simulink model "HSP_TC499_Trajectory_Planning_Control"  (R2025a)
settings: Solver=FixedStepAuto  StartTime=0.0  StopTime=SIM_TIME  FixedStep=0.01  RelTol=1e-3  EnableMultiTasking=on
values from neighbouring files (symbols this model uses):
  D_COEFF = 2.631    [init_PID_controller.m]
  I_COEFF = 4.2108    [init_PID_controller.m]
  P_COEFF = 9.4365    [init_PID_controller.m]
settings Model: Creator=chmurski  LastModifiedBy=MarikL
settings SolverCC: PositivePriorityOrder=on  AutoInsertRateTranBlk=on
settings OptimizationCC: OptimizeBlockIOStorage=off  BufferReuse=off  ReuseModelBlockBuffer=off  GlobalBufferReuse=off  ExpressionFolding=off  EnableMemcpy=off  PassReuseOutputArgsAs=Individual arguments  LocalBlockOutputs=off  ZeroExternalMemoryAtStartup=off  ZeroInternalMemoryAtStartup=off  MaxStackSize=2048  OptimizeDataStoreBuffers=off  BusAssignmentInplaceUpdate=off  OptimizationLevel=level0  OptimizationCustomize=off  EfficientTunableParamExpr=on
settings DebuggingCC: ParameterTunabilityLossMsg=error
settings HardwareCC: ProdBitPerPointer=32.0  ProdBitPerSizeT=32.0  ProdBitPerPtrDiffT=32.0  ProdLargestAtomicInteger=Long  ProdWordSize=32.0  ProdLongLongMode=on  ProdHWDeviceType=Infineon->TriCore
settings SFSimCC: MATLABDynamicMemAlloc=off
settings RTWCC: SystemTargetFile=ert.tlc  HardwareBoard=Infineon AURIX TC4x - TriBoards  GenCodeOnly=on  PackageGeneratedCodeAndArtifacts=on  PackageName=packaged_code  TemplateMakefile=ert_default_tmf  Toolchain=TASKING SmartCode for TriCore  BuildConfiguration=Debug  GPUComputeCapability=3.5  Description=Embedded Coder
settings CodeAppCC: ForceParamTrailComments=on  IgnoreCustomStorageClasses=off  MaxIdLength=256.0  OperatorAnnotations=on  SimulinkDataObjDesc=on  SFDataObjDesc=on  InsertBlockDesc=on
settings ERTTargetCC: ExtModeTransport=0.0  ExtModeStaticAlloc=off  ExtModeMexFile=ext_comm  ExtModeIntrfLevel=Level1  InlinedParameterPlacement=Hierarchical  DynamicArrayContainerType=coder::array  SupportContinuousTime=on  SupportVariableSizeSignals=on  ParenthesesLevel=Minimum

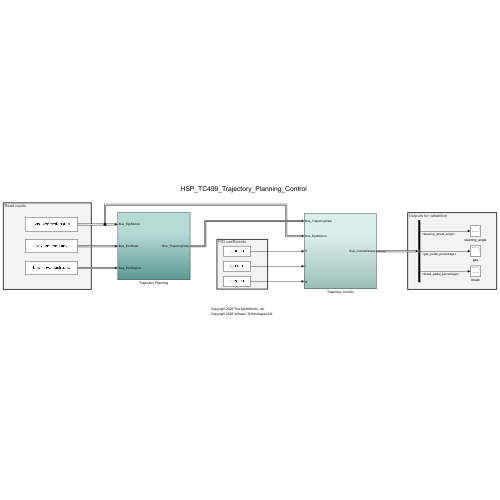
[thumbnail: Simulink's stored preview of the top-level diagram]
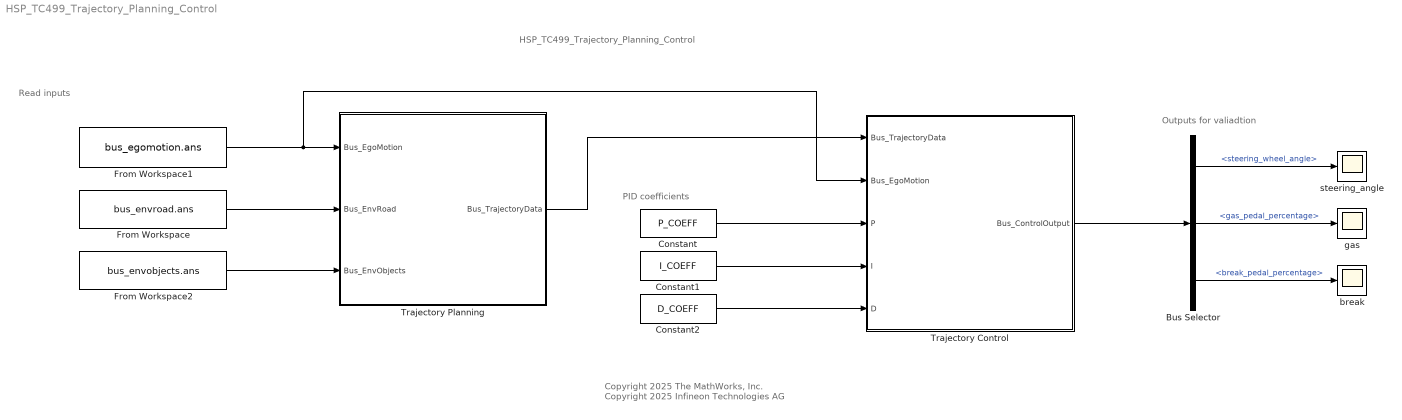
== system HSP_TC499_Trajectory_Planning_Control ==
  note: Copyright 2025 The MathWorks, Inc.
      | Copyright 2025 Infineon Technologies AG
  note: PID coefficients
  note: Read inputs
  note: Outputs for valiadtion
  note: HSP_TC499_Trajectory_Planning_Control
  Bus Selector : BusSelector  OutputSignals=steering_wheel_angle,gas_pedal_percentage,break_pedal_percentage
  Constant : Constant  Value=P_COEFF  OutDataTypeStr=single
  Constant1 : Constant  Value=I_COEFF  OutDataTypeStr=single
  Constant2 : Constant  Value=D_COEFF  OutDataTypeStr=single
  From Workspace : FromWorkspace  VariableName=bus_envroad.ans  OutDataTypeStr=Bus: Bus_EnvRoad  SampleTime=0.01  Interpolate=off  OutputAfterFinalValue=Setting to zero
  From Workspace1 : FromWorkspace  VariableName=bus_egomotion.ans  OutDataTypeStr=Bus: Bus_EgoMotion  SampleTime=0.01  Interpolate=off  OutputAfterFinalValue=Setting to zero
  From Workspace2 : FromWorkspace  VariableName=bus_envobjects.ans  OutDataTypeStr=Bus: Bus_EnvObjects  SampleTime=0.01  Interpolate=off  OutputAfterFinalValue=Setting to zero
  Trajectory Control : Subsystem
  Trajectory Planning : Subsystem
  break : Scope
      settings: ActiveDisplayYMinimum=0.90787  ActiveDisplayYMaximum=1.5513
  gas : Scope
      settings: ActiveDisplayYMinimum=-1  ActiveDisplayYMaximum=1  DataLoggingVariableName=ScopeData2
  steering_angle : Scope
      settings: ActiveDisplayYMinimum=-0.37276  ActiveDisplayYMaximum=0.98681
  wires:
  Trajectory Planning/1(Bus_TrajectoryData) -> Trajectory Control/1(Bus_TrajectoryData)
  From Workspace1/1 -> Trajectory Control/2(Bus_EgoMotion), Trajectory Planning/1(Bus_EgoMotion)
  From Workspace/1 -> Trajectory Planning/2(Bus_EnvRoad)
  From Workspace2/1 -> Trajectory Planning/3(Bus_EnvObjects)
  Constant/1 -> Trajectory Control/3(P)
  Constant1/1 -> Trajectory Control/4(I)
  Constant2/1 -> Trajectory Control/5(D)
  Trajectory Control/1(Bus_ControlOutput) -> Bus Selector/1
  Bus Selector/1 -> steering_angle/1  "<steering_wheel_angle>"
  Bus Selector/2 -> gas/1  "<gas_pedal_percentage>"
  Bus Selector/3 -> break/1  "<break_pedal_percentage>"

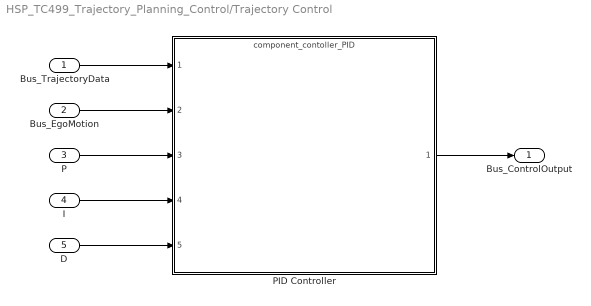
== system HSP_TC499_Trajectory_Planning_Control/Trajectory Control ==
  Bus_TrajectoryData : Inport
  Bus_EgoMotion : Inport  Port=2
  P : Inport  Port=3
  I : Inport  Port=4
  D : Inport  Port=5
  PID Controller : ModelReference  ModelNameDialog=component_contoller_PID.slx  SimulationMode=Normal  ModelReferenceVersion=10.0
  Bus_ControlOutput : Outport
  wires:
  PID Controller/1 -> Bus_ControlOutput/1
  Bus_TrajectoryData/1 -> PID Controller/1
  Bus_EgoMotion/1 -> PID Controller/2
  P/1 -> PID Controller/3
  I/1 -> PID Controller/4
  D/1 -> PID Controller/5

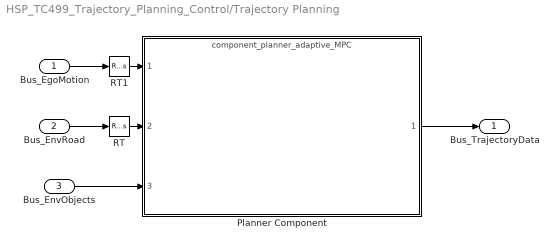
== system HSP_TC499_Trajectory_Planning_Control/Trajectory Planning ==
  Bus_EgoMotion : Inport  OutDataTypeStr=Bus: Bus_EgoMotion
  Bus_EnvRoad : Inport  Port=2  OutDataTypeStr=Bus: Bus_EnvRoad
  Bus_EnvObjects : Inport  Port=3  OutDataTypeStr=Bus: Bus_EnvObjects
  Planner Component : ModelReference  ModelNameDialog=component_planner_adaptive_MPC.slx  SimulationMode=Normal  ModelReferenceVersion=16.1
  RT : RateTransition
  RT1 : RateTransition
  Bus_TrajectoryData : Outport  OutDataTypeStr=Bus: Bus_TrajectoryData  VectorParamsAs1DForOutWhenUnconnected=off
  wires:
  Bus_EgoMotion/1 -> RT1/1
  Bus_EnvRoad/1 -> RT/1
  Bus_EnvObjects/1 -> Planner Component/3
  Planner Component/1 -> Bus_TrajectoryData/1
  RT/1 -> Planner Component/2
  RT1/1 -> Planner Component/1
